simulink model "myScanerAPIControl_SMC_v2_2"  (R2017a)
settings: Solver=FixedStepDiscrete  StartTime=0.0  StopTime=inf  RelTol=1e-3  EnableMultiTasking=on
undefined symbols (not defined in the file): a1, a2, a3, alpha, beta, DiscIntNeverNeededParam, lambda, magnitude
libraries: SCANeR_API x13
settings Model: Creator=alepicard  LastModifiedBy=Vittorio Sanchez
settings DataIOCC: LimitDataPoints=on  SaveFormat=Array  SignalLoggingSaveFormat=ModelDataLogs
settings OptimizationCC: ExpressionDepthLimit=2147483647  InitFltsAndDblsToZero=on
settings DebuggingCC: UnderspecifiedInitializationDetection=Classic  MergeDetectMultiDrivingBlocksExec=none  SolverPrmCheckMsg=warning  FcnCallInpInsideContextMsg=warning  StateNameClashWarn=warning  SFUnexpectedBacktrackingDiag=warning  SFNoUnconditionalDefaultTransitionDiag=warning  SFExecutionAtInitializationDiag=none
settings HardwareCC: ProdBitPerPointer=32  ProdBitPerSizeT=32  ProdBitPerPtrDiffT=32  ProdLargestAtomicFloat=None  ProdIntDivRoundTo=Undefined  ProdEndianess=Unspecified  ProdWordSize=32  ProdHWDeviceType=32-bit Generic
settings ModelReferenceCC: PropagateSignalLabelsOutOfModel=off
settings RTWCC: SystemTargetFile=grt_scanerapi.tlc  TemplateMakefile=grt_scanerapi_vc.tmf  Description=SCANeR API Real-Time Target
settings STFCustomTargetCC: CombineOutputUpdateFcns=on  MatFileLogging=on  GRTInterface=off  SystemTargetFile=grt_scanerapi.tlc
settings GRTTargetCC: TargetLangStandard=C89/C90 (ANSI)  ParMdlRefBuildCompliant=off  CompOptLevelCompliant=off  ConcurrentExecutionCompliant=off  CPPClassGenCompliant=off  UseToolchainInfoCompliant=off
settings ConfigComp: CovMetricSettings=dw  CovHtmlReporting=on  CovSaveCumulativeToWorkspaceVar=on  CovSaveSingleToWorkspaceVar=on  CovExternalEMLEnable=off

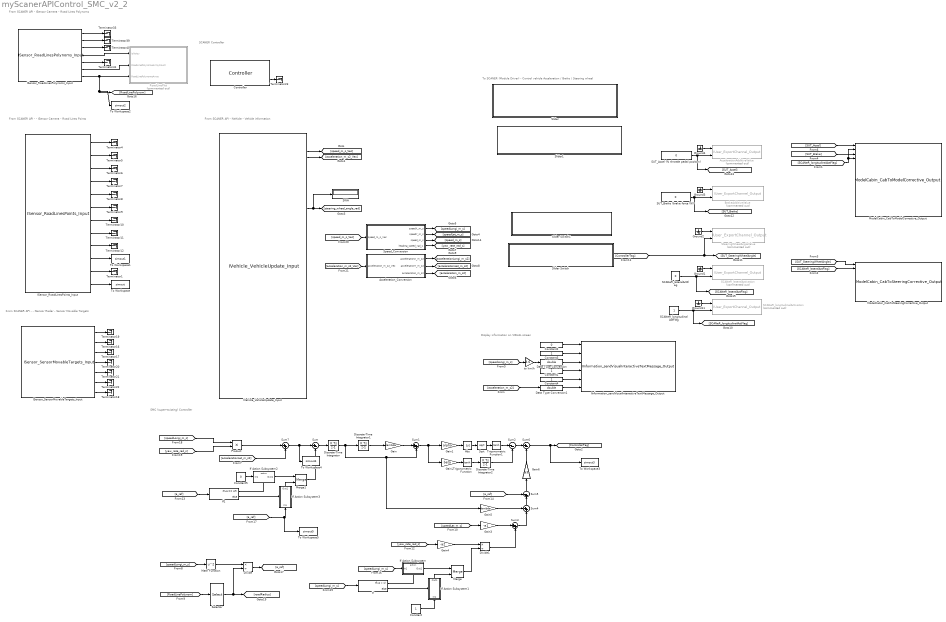
== system myScanerAPIControl_SMC_v2_2 ==
  note: SCANER Controller
  note: From SCANER API - IVehicle - Vehicle information
  note: To SCANER (Module Driver) - Control vehicle Acceleration / Brake / Steering wheel
  note: Display information on VISUAL screen
  note: From SCANER API - ISensor Camera
      |  - Road Lines Polynoms
  note: From SCANER API -  - ISensor Camera
      | - Road Lines Points
  note: From SCANER API -  - ISensor Radar -
      | Sensor Movable Targets
  note: SMC (super-twisting) Controller
  Abs : Abs
  AccelerationAdditiveValue : SCANeR_API/Network outputs/IUser/IUser_ExportChannel_Output  Priority=2  Commented=on  no=20
  Acceleration_Conversion : Subsystem  TreatAsAtomicUnit=on
  BrakeAdditiveValue : SCANeR_API/Network outputs/IUser/IUser_ExportChannel_Output  Priority=2  Commented=on  no=21
  Constant : Constant
  Constant1 : Constant  VectorParams1D=off  SampleTime=-1
  Constant2 : Constant  Value=0  VectorParams1D=off  SampleTime=-1
  Constant3 : Constant  VectorParams1D=off  SampleTime=-1
  Constant4 : Constant  VectorParams1D=off  SampleTime=-1
  Constant5 : Constant  Value=0
  Controller : SCANeR_API/Controller  Priority=1  Config='vitto_config'  ProcName='SIMULINK'  Frequency=100  NetworkOutputFrequency=10  TimeOut=30  IsSynchronized=on
  Data Type Conversion : DataTypeConversion  OutDataTypeStr=double
  Data Type Conversion1 : DataTypeConversion  OutDataTypeStr=double
  Discrete-Time Integrator : DiscreteIntegrator  InitialConditionSetting=State (most efficient)  SampleTime=-1  ICPrevOutput=DiscIntNeverNeededParam  ICPrevScaledInput=DiscIntNeverNeededParam
  Discrete-Time Integrator1 : DiscreteIntegrator  InitialConditionSetting=State (most efficient)  SampleTime=-1  ICPrevOutput=DiscIntNeverNeededParam  ICPrevScaledInput=DiscIntNeverNeededParam
  Discrete-Time Integrator2 : DiscreteIntegrator  InitialConditionSetting=State (most efficient)  SampleTime=-1  ICPrevOutput=DiscIntNeverNeededParam  ICPrevScaledInput=DiscIntNeverNeededParam
  Divide : Product  Inputs=*/
  Divide1 : Product  Inputs=*/
  Gain : Gain  Gain=lambda
  Gain1 : Gain  Gain=alpha
  Gain2 : Gain  Gain=beta
  Gain3 : Gain  Gain=-a1
  Gain4 : Gain  Gain=-a2
  Gain5 : Gain  Gain=lambda
  Gain6 : Gain  Gain=a3
  Ground{1..4,11} (5 alike) : Ground
  IInformation_sendVisualInteractiveTextMessage_Output : SCANeR_API/Network outputs/IInformation/IInformation_sendVisualInteractiveTextMessage_Output  Priority=2  beginString='Speed (km/h): '  middleString=''  endString='Accel (m/s): '  displayAreaName='LEFT'
  ISensor_RoadLinesPoints_Input : SCANeR_API/Network inputs/ISensor/ISensor_RoadLinesPoints_Input  Priority=2  ev=off  globalId=0100000
  ISensor_RoadLinesPolynoms_Input : SCANeR_API/Network inputs/ISensor/ISensor_RoadLinesPolynoms_Input  Priority=2  ev=off  globalId=0100000
  ISensor_SensorMovableTargets_Input : SCANeR_API/Network inputs/ISensor/ISensor_SensorMovableTargets_Input  Priority=2  ev=on  globalId=0300000
  IVehicle_VehicleUpdate_Input : SCANeR_API/Network inputs/IVehicle/IVehicle_VehicleUpdate_Input  Priority=2  ev=off  vhlId=0
  If : If  IfExpression=u1 > 1
  If Action Subsystem : Subsystem  TreatAsAtomicUnit=on
  If Action Subsystem1 : Subsystem  TreatAsAtomicUnit=on
  If Action Subsystem2 : Subsystem  TreatAsAtomicUnit=on
  If Action Subsystem3 : Subsystem  TreatAsAtomicUnit=on
  If1 : If  IfExpression=u1 == inf
  Math Function : Math  Operator=square  SaturateOnIntegerOverflow=on
  Merge : Merge
  Merge1 : Merge
  ModelCabin_CabToModelCorrective_Output : SCANeR_API/SHM outputs/ModelCabin/ModelCabin_CabToModelCorrective_Output  Priority=2  shmId=0
  ModelCabin_CabToSteeringCorrective_Output : SCANeR_API/SHM outputs/ModelCabin/ModelCabin_CabToSteeringCorrective_Output  Priority=2  shmId=0
  Product : Product
  RoadLinePlot : MATLAB Function  Commented=on  TreatAsAtomicUnit=on
  SCANeR_lateralActFlag : Constant  Value=0
  SCANeR_lateralActivation : SCANeR_API/Network outputs/IUser/IUser_ExportChannel_Output  Priority=2  Commented=on  no=23
  SCANeR_longitudinalActFlag : Constant
  SCANeR_longitudinalActivation : SCANeR_API/Network outputs/IUser/IUser_ExportChannel_Output  Priority=2  Commented=on  no=24
  SUT_Accel (% throttle pedal position) : Constant  Value=0
  SUT_Brake (brake force (N)) : Constant  Value=0
  SWA : Display
  Selector : Selector  InputPortWidth=1792  IndexOptions=Index vector (dialog)  Indices=[7]  OutputSizes=1
  Slider : Subsystem  DialogController=hmiCreateDDGDialog  IsWebBlock=on  mask(MWDashboardBlock){webBlockId=258a6095-db8d-43df-809a-c74485d0d6d2, webBlockType=slider, ShowInLibBrowser=on, ShowInitialText=on, HMISrcModelName=myScanerAPIControl_SMC_v2_2}
      mask prompts: webBlockId "WebBlock Id"; webBlockType "WebBlock Type"; HMISrcModelName "Source Model"
      mask help: SimulinkHMI:dialogs:SliderDialogDesc
      mask Help: helpview([docroot '/mapfiles/simulink.map'], 'hmi_slider')
      mask Display:
      | if strcmp(get_param(bdroot(gcb),'BlockDiagramType'), 'library')
      |     image([(matlabroot) '/toolbox/simulink/hmi/icons/Slider.png']);
      | end
  Slider Switch : Subsystem  DialogController=hmiCreateDDGDialog  IsWebBlock=on  mask(MWDashboardBlock){webBlockId=2fac1965-2567-4f0f-8ac3-e04a12885fb9, webBlockType=sliderswitch, ShowInLibBrowser=on, ShowInitialText=on, HMISrcModelName=myScanerAPIControl_SMC_v2_2}
      mask prompts: webBlockId "WebBlock Id"; webBlockType "WebBlock Type"; HMISrcModelName "Source Model"
      mask help: SimulinkHMI:dialogs:SwitchDialogDesc
      mask Help: helpview([docroot '/mapfiles/simulink.map'], 'hmi_slider_switch')
      mask Display:
      | if strcmp(get_param(bdroot(gcb),'BlockDiagramType'), 'library')
      |     image([(matlabroot) '/toolbox/simulink/hmi/icons/SliderSwitch.png']);
      | end
  Slider Switch1 : Subsystem  DialogController=hmiCreateDDGDialog  IsWebBlock=on  mask(MWDashboardBlock){webBlockId=0c6f8257-7b8c-4f8b-ae78-f20602ab88ff, webBlockType=sliderswitch, ShowInLibBrowser=on, ShowInitialText=on, HMISrcModelName=myScanerAPIControl_SMC_v2_2}
      mask prompts: webBlockId "WebBlock Id"; webBlockType "WebBlock Type"; HMISrcModelName "Source Model"
      mask help: SimulinkHMI:dialogs:SwitchDialogDesc
      mask Help: helpview([docroot '/mapfiles/simulink.map'], 'hmi_slider_switch')
      mask Display:
      | if strcmp(get_param(bdroot(gcb),'BlockDiagramType'), 'library')
      |     image([(matlabroot) '/toolbox/simulink/hmi/icons/SliderSwitch.png']);
      | end
  Slider1 : Subsystem  DialogController=hmiCreateDDGDialog  IsWebBlock=on  mask(MWDashboardBlock){webBlockId=86d26918-d391-4a58-ba15-344714f27837, webBlockType=slider, ShowInLibBrowser=on, ShowInitialText=on, HMISrcModelName=myScanerAPIControl_SMC_v2_2}
      mask prompts: webBlockId "WebBlock Id"; webBlockType "WebBlock Type"; HMISrcModelName "Source Model"
      mask help: SimulinkHMI:dialogs:SliderDialogDesc
      mask Help: helpview([docroot '/mapfiles/simulink.map'], 'hmi_slider')
      mask Display:
      | if strcmp(get_param(bdroot(gcb),'BlockDiagramType'), 'library')
      |     image([(matlabroot) '/toolbox/simulink/hmi/icons/Slider.png']);
      | end
  Speed_Conversion : Subsystem  TreatAsAtomicUnit=on
  Sqrt : Sqrt  SaturateOnIntegerOverflow=on
  SteeringWheelAngleValue : SCANeR_API/Network outputs/IUser/IUser_ExportChannel_Output  Priority=2  Commented=on  no=22
  Sum : Sum  Inputs=|+-
  Sum1 : Sum  Inputs=|++
  Sum2 : Sum  Inputs=|--
  Sum3 : Sum  Inputs=|++
  Sum4 : Sum  Inputs=++|
  Sum5 : Sum  Inputs=-+|
  Sum6 : Sum  Inputs=|+-
  Sum7 : Sum  Inputs=|++
  Terminator{1,4..12,16..23,33,39..41} (22 alike) : Terminator
  To Workspace : ToWorkspace  VariableName=simout  SaveFormat=Timeseries  SampleTime=-1
  To Workspace1 : ToWorkspace  VariableName=simout1  SaveFormat=Timeseries  SampleTime=-1
  To Workspace2 : ToWorkspace  VariableName=simout2  SaveFormat=Timeseries  SampleTime=-1
  To Workspace3 : ToWorkspace  VariableName=simout3  SaveFormat=Timeseries  SampleTime=-1
  To Workspace4 : ToWorkspace  VariableName=simout4  SaveFormat=Timeseries  SampleTime=-1
  To Workspace5 : ToWorkspace  VariableName=simout5  SaveFormat=Timeseries  SampleTime=-1
  Trigonometric Function : Trigonometry  Operator=tanh
  Trigonometric Function1 : Trigonometry  Operator=tanh
  to km/h : Gain  Gain=3.6
  wires:
  Controller/2 -> Terminator23/1
  Constant2/1 -> IInformation_sendVisualInteractiveTextMessage_Output/1
  Data Type Conversion/1 -> IInformation_sendVisualInteractiveTextMessage_Output/3
  Constant3/1 -> IInformation_sendVisualInteractiveTextMessage_Output/2
  [speedLongi_m_s] -> to km/h/1
  IVehicle_VehicleUpdate_Input/14 -> [steering_wheel_angle_rad], SWA/1
  Speed_Conversion/3(speed_m_s) -> [speed_m_s]
  Acceleration_Conversion/3(acceleration_m_s2) -> [acceleration_m_s2]
  [speed_m_s_Vec] -> Speed_Conversion/1(speed_m_s_Vec)
  [acceleration_m_s2_Vec] -> Acceleration_Conversion/1(acceleration_m_s2_Vec)
  IVehicle_VehicleUpdate_Input/5 -> [acceleration_m_s2_Vec]
  IVehicle_VehicleUpdate_Input/4 -> [speed_m_s_Vec]
  Ground4/1 -> AccelerationAdditiveValue/1
  Speed_Conversion/2(speedY_m_s) -> [speedLat_m_s]
  Speed_Conversion/1(speedX_m_s) -> [speedLongi_m_s]
  Acceleration_Conversion/2(accelerationY_m_s2) -> [accelerationLat_m_s2]
  Acceleration_Conversion/1(accelerationX_m_s2) -> [accelerationLongi_m_s2]
  Ground3/1 -> BrakeAdditiveValue/1
  Ground2/1 -> SteeringWheelAngleValue/1
  Ground1/1 -> SCANeR_lateralActivation/1
  Ground11/1 -> SCANeR_longitudinalActivation/1
  SCANeR_longitudinalActFlag/1 -> [SCANeR_longitudinalActFlag], SCANeR_longitudinalActivation/2
  SCANeR_lateralActFlag/1 -> [SCANeR_lateralActFlag], SCANeR_lateralActivation/2
  SUT_Accel (% throttle pedal position)/1 -> [SUT_Accel], AccelerationAdditiveValue/2
  SUT_Brake (brake force (N))/1 -> [SUT_Brake], BrakeAdditiveValue/2
  to km/h/1 -> Data Type Conversion/1
  Constant1/1 -> IInformation_sendVisualInteractiveTextMessage_Output/4
  Constant4/1 -> IInformation_sendVisualInteractiveTextMessage_Output/5
  Data Type Conversion1/1 -> IInformation_sendVisualInteractiveTextMessage_Output/6
  [acceleration_m_s2] -> Data Type Conversion1/1
  ISensor_RoadLinesPolynoms_Input/7 -> To Workspace2/1, [RoadLinePolynom], RoadLinePlot/3(RoadLinePolynomeArray)
  ISensor_RoadLinesPolynoms_Input/6 -> RoadLinePlot/2(RoadLinePolynomeArrayCount)
  ISensor_RoadLinesPolynoms_Input/4 -> RoadLinePlot/1(isNoisy)
  ISensor_RoadLinesPolynoms_Input/1 -> Terminator33/1
  ISensor_RoadLinesPolynoms_Input/2 -> Terminator39/1
  ISensor_RoadLinesPolynoms_Input/3 -> Terminator40/1
  ISensor_RoadLinesPolynoms_Input/5 -> Terminator41/1
  ISensor_RoadLinesPoints_Input/1 -> Terminator4/1
  ISensor_RoadLinesPoints_Input/2 -> Terminator5/1
  ISensor_RoadLinesPoints_Input/3 -> Terminator6/1
  ISensor_RoadLinesPoints_Input/4 -> Terminator7/1
  ISensor_RoadLinesPoints_Input/5 -> Terminator8/1
  ISensor_RoadLinesPoints_Input/6 -> Terminator9/1
  ISensor_RoadLinesPoints_Input/7 -> Terminator10/1
  ISensor_RoadLinesPoints_Input/8 -> Terminator11/1
  ISensor_RoadLinesPoints_Input/9 -> Terminator12/1
  ISensor_RoadLinesPoints_Input/10 -> To Workspace1/1
  ISensor_RoadLinesPoints_Input/11 -> Terminator1/1
  ISensor_RoadLinesPoints_Input/12 -> To Workspace/1
  ISensor_SensorMovableTargets_Input/4 -> Terminator20/1
  ISensor_SensorMovableTargets_Input/5 -> Terminator21/1
  ISensor_SensorMovableTargets_Input/6 -> Terminator22/1
  ISensor_SensorMovableTargets_Input/3 -> Terminator17/1
  ISensor_SensorMovableTargets_Input/2 -> Terminator16/1
  ISensor_SensorMovableTargets_Input/1 -> Terminator19/1
  ISensor_SensorMovableTargets_Input/7 -> Terminator18/1
  [SCANeR_lateralActFlag] -> ModelCabin_CabToSteeringCorrective_Output/2
  [SCANeR_longitudinalActFlag] -> ModelCabin_CabToModelCorrective_Output/2, ModelCabin_CabToModelCorrective_Output/4
  [SUT_SteeringWheelAngle] -> ModelCabin_CabToSteeringCorrective_Output/1
  [SUT_Brake] -> ModelCabin_CabToModelCorrective_Output/3
  [SUT_Accel] -> ModelCabin_CabToModelCorrective_Output/1
  Sum/1 -> Discrete-Time Integrator/1
  Gain/1 -> Sum1/1
  Sum1/1 -> Gain2/1, Gain1/1
  Gain1/1 -> Abs/1
  Abs/1 -> Sqrt/1
  Sqrt/1 -> Trigonometric Function1/1
  Gain2/1 -> Trigonometric Function/1
  Trigonometric Function/1 -> Discrete-Time Integrator2/1
  Trigonometric Function1/1 -> Sum2/1
  [speedLongi_m_s] -> Math Function/1
  [RoadLinePolynom] -> Selector/1
  Math Function/1 -> Divide/1
  Selector/1 -> [roadRadius], Divide/2
  Divide/1 -> [a_ref]
  Discrete-Time Integrator/1 -> Discrete-Time Integrator1/1, Gain5/1, Sum1/2
  Discrete-Time Integrator1/1 -> Gain/1
  Discrete-Time Integrator2/1 -> Sum2/2
  [ControllerTag] -> SteeringWheelAngleValue/2, [SUT_SteeringWheelAngle]
  [speedLat_m_s] -> Gain3/1
  [yaw_rate_rad_s] -> Gain4/1
  Gain3/1 -> Sum3/1
  Sum3/1 -> Sum4/2
  Gain5/1 -> Sum4/1
  [a_ref] -> Sum5/1
  Sum4/1 -> Sum5/2
  Sum5/1 -> Gain6/1
  Sum2/1 -> Sum6/1
  Sum6/1 -> To Workspace3/1, [ControllerTag]
  Gain6/1 -> Sum6/2
  Gain4/1 -> Divide1/1
  Divide1/1 -> Sum3/2
  Speed_Conversion/4(heading_speed_rad_s) -> [yaw_rate_rad_s]
  [speedLongi_m_s] -> If/1
  If/1 -> If Action Subsystem/Action
  If/2 -> If Action Subsystem1/Action
  [speedLongi_m_s] -> If Action Subsystem/1(In1)
  If Action Subsystem/1(Out1) -> Merge/1
  If Action Subsystem1/1(Out1) -> Merge/2
  Merge/1 -> Divide1/2
  Constant/1 -> If Action Subsystem1/1(In1)
  Constant5/1 -> If Action Subsystem2/1(In1)
  If1/1 -> If Action Subsystem2/Action
  [a_ref] -> To Workspace5/1, If Action Subsystem3/1(In1)
  [a_ref] -> If1/1
  If Action Subsystem3/1(Out1) -> Merge1/2
  If1/2 -> If Action Subsystem3/Action
  If Action Subsystem2/1(Out1) -> Merge1/1
  Merge1/1 -> Sum/2
  Sum7/1 -> To Workspace4/1, Sum/1
  [accelerationLat_m_s2] -> Sum7/2
  [speedLongi_m_s] -> Product/1
  [yaw_rate_rad_s] -> Product/2
  Product/1 -> Sum7/1

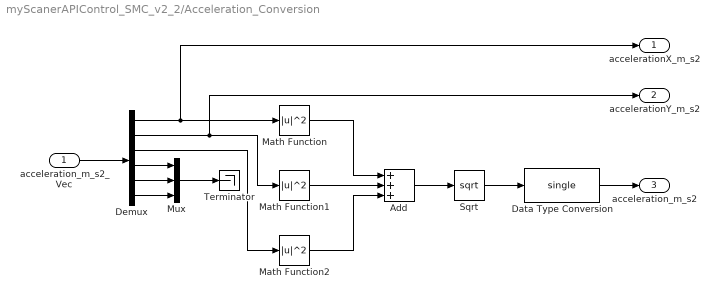
== system myScanerAPIControl_SMC_v2_2/Acceleration_Conversion ==
  acceleration_m_s2_Vec : Inport
      settings: AttributesFormatString=%<OutDataTypeStr>
  Add : Sum  Inputs=+++
  Data Type Conversion : DataTypeConversion  OutDataTypeStr=single
  Demux : Demux  Outputs=6
  Math Function : Math  Operator=magnitude^2  SaturateOnIntegerOverflow=on
  Math Function1 : Math  Operator=magnitude^2  SaturateOnIntegerOverflow=on
  Math Function2 : Math  Operator=magnitude^2  SaturateOnIntegerOverflow=on
  Mux : Mux  Inputs=3
  Sqrt : Sqrt  SaturateOnIntegerOverflow=on
  Terminator : Terminator
  accelerationX_m_s2 : Outport
      settings: AttributesFormatString=%<OutDataTypeStr>
  accelerationY_m_s2 : Outport  Port=2
      settings: AttributesFormatString=%<OutDataTypeStr>
  acceleration_m_s2 : Outport  Port=3
      settings: AttributesFormatString=%<OutDataTypeStr>
  wires:
  acceleration_m_s2_Vec/1 -> Demux/1
  Demux/3 -> Math Function2/1
  Demux/2 -> accelerationY_m_s2/1, Math Function1/1
  Demux/1 -> accelerationX_m_s2/1, Math Function/1
  Sqrt/1 -> Data Type Conversion/1
  Add/1 -> Sqrt/1
  Math Function2/1 -> Add/3
  Math Function1/1 -> Add/2
  Math Function/1 -> Add/1
  Data Type Conversion/1 -> acceleration_m_s2/1
  Demux/4 -> Mux/1
  Demux/5 -> Mux/2
  Demux/6 -> Mux/3
  Mux/1 -> Terminator/1

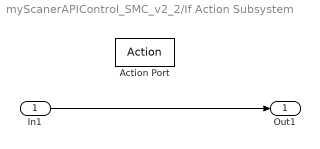
== system myScanerAPIControl_SMC_v2_2/If Action Subsystem ==
  In1 : Inport
  Action Port : ActionPort  ActionType=then
  Out1 : Outport
  wires:
  In1/1 -> Out1/1

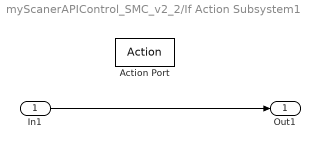
== system myScanerAPIControl_SMC_v2_2/If Action Subsystem1 ==
  In1 : Inport
  Action Port : ActionPort  ActionType=else
  Out1 : Outport
  wires:
  In1/1 -> Out1/1

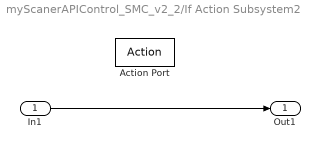
== system myScanerAPIControl_SMC_v2_2/If Action Subsystem2 ==
  In1 : Inport
  Action Port : ActionPort  ActionType=then
  Out1 : Outport
  wires:
  In1/1 -> Out1/1

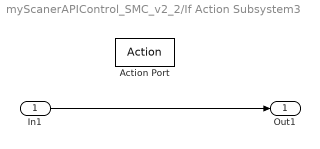
== system myScanerAPIControl_SMC_v2_2/If Action Subsystem3 ==
  In1 : Inport
  Action Port : ActionPort  ActionType=else
  Out1 : Outport
  wires:
  In1/1 -> Out1/1

== system myScanerAPIControl_SMC_v2_2/Slider ==

== system myScanerAPIControl_SMC_v2_2/Slider Switch ==

== system myScanerAPIControl_SMC_v2_2/Slider Switch1 ==

== system myScanerAPIControl_SMC_v2_2/Slider1 ==

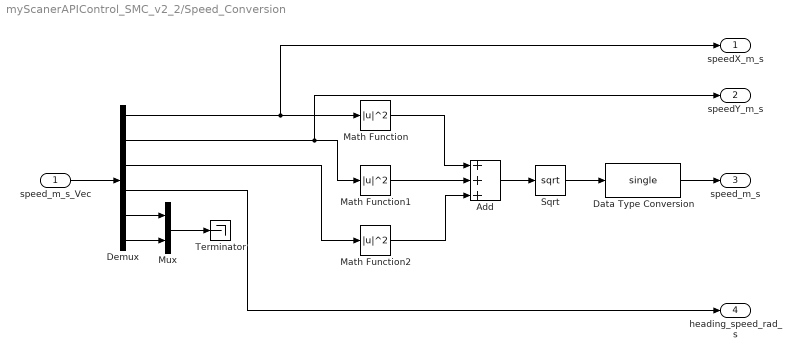
== system myScanerAPIControl_SMC_v2_2/Speed_Conversion ==
  speed_m_s_Vec : Inport
      settings: AttributesFormatString=%<OutDataTypeStr>
  Add : Sum  Inputs=+++
  Data Type Conversion : DataTypeConversion  OutDataTypeStr=single
  Demux : Demux  Outputs=6
  Math Function : Math  Operator=magnitude^2  SaturateOnIntegerOverflow=on
  Math Function1 : Math  Operator=magnitude^2  SaturateOnIntegerOverflow=on
  Math Function2 : Math  Operator=magnitude^2  SaturateOnIntegerOverflow=on
  Mux : Mux  Inputs=2
  Sqrt : Sqrt  SaturateOnIntegerOverflow=on
  Terminator : Terminator
  speedX_m_s : Outport
      settings: AttributesFormatString=%<OutDataTypeStr>
  speedY_m_s : Outport  Port=2
      settings: AttributesFormatString=%<OutDataTypeStr>
  speed_m_s : Outport  Port=3
      settings: AttributesFormatString=%<OutDataTypeStr>
  heading_speed_rad_s : Outport  Port=4
      settings: AttributesFormatString=%<OutDataTypeStr>
  wires:
  Demux/1 -> speedX_m_s/1, Math Function/1
  Math Function1/1 -> Add/2
  Math Function2/1 -> Add/3
  Add/1 -> Sqrt/1
  Sqrt/1 -> Data Type Conversion/1
  Demux/2 -> speedY_m_s/1, Math Function1/1
  Demux/3 -> Math Function2/1
  Demux/6 -> Mux/2
  speed_m_s_Vec/1 -> Demux/1
  Data Type Conversion/1 -> speed_m_s/1
  Math Function/1 -> Add/1
  Mux/1 -> Terminator/1
  Demux/5 -> Mux/1
  Demux/4 -> heading_speed_rad_s/1

== matlab function myScanerAPIControl_SMC_v2_2/RoadLinePlot ==
  data: isNoisy input; RoadLinePolynomeArrayCount input; RoadLinePolynomeArray input
function fcn(isNoisy,RoadLinePolynomeArrayCount, RoadLinePolynomeArray)

%coder.extrinsic('cell')

% Init
nbPoints = 21;
length = 7;
RoadLineArray = zeros(10,length);
lineCoef = zeros(10,4);
YLat = zeros(nbPoints,2);

if (isNoisy == false && RoadLinePolynomeArrayCount>0)
    
    % loop on detected lines, from most left to most right lines
    for n=1:RoadLinePolynomeArrayCount
        RoadLineArray(n,1) = RoadLinePolynomeArray(1+(n-1)*length);
        RoadLineArray(n,2) = RoadLinePolynomeArray(2+(n-1)*length);
        RoadLineArray(n,3) = RoadLinePolynomeArray(3+(n-1)*length);
        RoadLineArray(n,4) = RoadLinePolynomeArray(4+(n-1)*length);
        RoadLineArray(n,5) = RoadLinePolynomeArray(5+(n-1)*length);
        RoadLineArray(n,6) = RoadLinePolynomeArray(6+(n-1)*length);
        RoadLineArray(n,7) = RoadLinePolynomeArray(7+(n-1)*length);
        
        % y = P(x) = c0 + c1*x + c2*x*x + c3*x*x*x
        lineCoef(n,1) = RoadLineArray(n,5); % c3
        lineCoef(n,2) = RoadLineArray(n,4); % c2
        lineCoef(n,3) = RoadLineArray(n,3); % c1
        lineCoef(n,4) = RoadLineArray(n,2); % c0

    end
    
    % Define longitudinal horizon
    XLong = linspace(0,20,nbPoints)';

    % Calculate the lateral deviation along the longitudinal horizon
    for n=1:2
        YLat(:,n) = polyval(lineCoef(RoadLinePolynomeArrayCount+1-n,:)',XLong);
    end
    
    % Plot 2 lines: right lines and left lines of the right lane.
    plot(YLat(:,1),XLong,'-b',YLat(:,2),XLong,'-r');
    hold off
    title('Lane marking [x,y] Ego referential');
    xlabel('LATERAL (m)'); % x-axis label
    ylabel('LONGITUDINAL (m)'); % y-axis label
    set(gca,'XDir','reverse');
    axis([-3 3 -0.5 20]);
    
    grid on; 
    grid minor;
    
end
